simulink model "Full_quadcopter_GR"  (Simulink 7.7)
settings: Solver=ode45  StartTime=0.0  StopTime=10.0  RelTol=1e-3
values from neighbouring files (symbols this model uses):
  b = 9.7575e-6    (= 9.7575e-06)    [ForcesTest.m]    (also in QuadDynamics.m = 9.937e-09; QuadDynamicsC.m = 1.7246e-06; Quadparameters.m = 3.13e-05; quadparam.m = 3.13e-05)
  g = 9.81    [ForcesTest.m]    (also in QuadDynamics.m; QuadDynamicsC.m; Quadparameters.m; quadparam.m)
  k = k+1    (= 1)    [ForcesTest.m]    (also in QuadDynamics.m = 3.82192307692e-10; QuadDynamicsC.m = 6.633e-08)
  m = 1.282    [ForcesTest.m]    (also in QuadDynamics.m = 1.284; QuadDynamicsC.m = 1.284; Quadparameters.m = 0.65; quadparam.m = 0.65)
undefined symbols (not defined in the file or in its folder): r1, r2
settings Model: Creator=Alexey  LastModifiedBy=Alexey

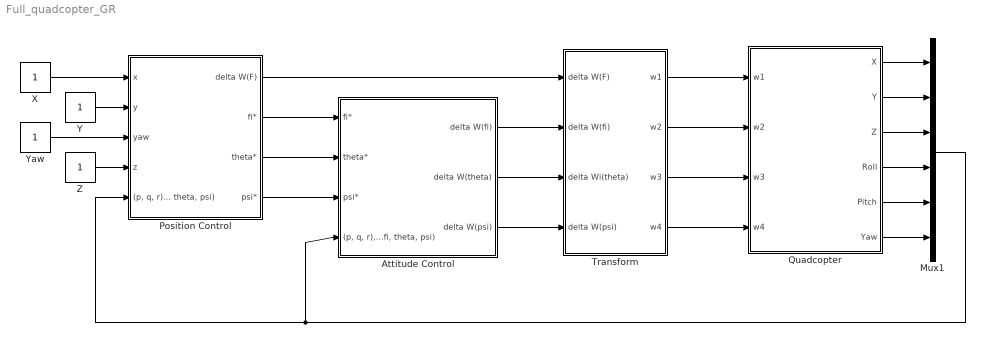
== system Full_quadcopter_GR ==
  Attitude Control : Subsystem
  Mux1 : Mux  Inputs=6
  Position Control : Subsystem
  Quadcopter : Subsystem
  Transform : Subsystem
  X : Constant
  Y : Constant
  Yaw : Constant
  Z : Constant
  wires:
  X/1 -> Position Control/1(x)
  Mux1/1 -> Attitude Control/4("(p, q, r), (fi, theta, psi)"), Position Control/5("(p, q, r), (fi, theta, psi)")
  Quadcopter/1(X) -> Mux1/1
  Quadcopter/2(Y) -> Mux1/2
  Quadcopter/3(Z) -> Mux1/3
  Transform/1(w1) -> Quadcopter/1(w1)
  Transform/2(w2) -> Quadcopter/2(w2)
  Transform/3(w3) -> Quadcopter/3(w3)
  Transform/4(w4) -> Quadcopter/4(w4)
  Position Control/1(delta W(F)) -> Transform/1(delta W(F))
  Attitude Control/1(delta W(fi)) -> Transform/2(delta W(fi))
  Attitude Control/2(delta W(theta)) -> Transform/3(delta Wi(theta))
  Attitude Control/3(delta W(psi)) -> Transform/4(delta W(psi))
  Position Control/2(fi*) -> Attitude Control/1(fi*)
  Position Control/3(theta*) -> Attitude Control/2(theta*)
  Position Control/4(psi*) -> Attitude Control/3(psi*)
  Y/1 -> Position Control/2(y)
  Yaw/1 -> Position Control/3(yaw)
  Z/1 -> Position Control/4(z)
  Quadcopter/4(Roll) -> Mux1/4
  Quadcopter/5(Pitch) -> Mux1/5
  Quadcopter/6(Yaw) -> Mux1/6

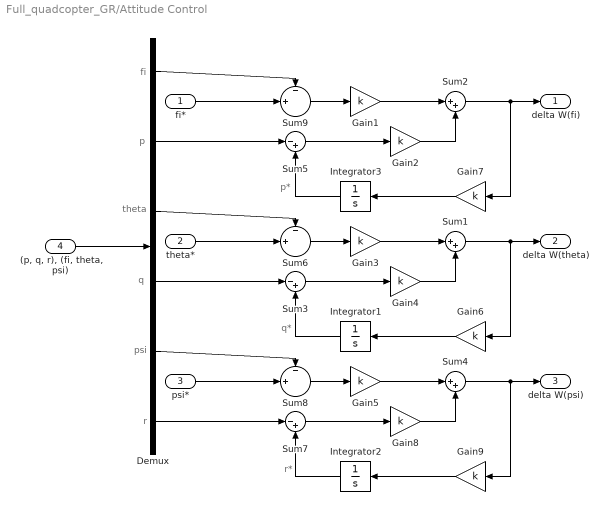
== system Full_quadcopter_GR/Attitude Control ==
  note: fi
  note: p
  note: theta
  note: q
  note: psi
  note: r
  note: q*
  note: p*
  note: r*
  fi* : Inport
  theta* : Inport  Port=2
  psi* : Inport  Port=3
  "(p, q, r), (fi, theta, psi)" : Inport  Port=4
  Demux : Demux  Outputs=6
  Gain{1..9} (9 alike) : Gain  Gain=k
  Integrator1 : Integrator
  Integrator2 : Integrator
  Integrator3 : Integrator
  Sum1 : Sum  Inputs=|++
  Sum2 : Sum  Inputs=|++
  Sum3 : Sum  Inputs=|-+
  Sum4 : Sum  Inputs=|++
  Sum5 : Sum  Inputs=|-+
  Sum6 : Sum  Inputs=-|+||
  Sum7 : Sum  Inputs=|-+
  Sum8 : Sum  Inputs=-|+||
  Sum9 : Sum  Inputs=-|+||
  delta W(fi) : Outport
  delta W(theta) : Outport  Port=2
  delta W(psi) : Outport  Port=3
  wires:
  psi*/1 -> Sum8/2
  Sum8/1 -> Gain5/1
  Gain5/1 -> Sum4/1
  "(p, q, r), (fi, theta, psi)"/1 -> Demux/1
  Sum7/1 -> Gain8/1
  Gain8/1 -> Sum4/2
  Gain9/1 -> Integrator2/1
  Integrator2/1 -> Sum7/2
  Demux/6 -> Sum7/1
  Demux/5 -> Sum8/1
  Sum4/1 -> delta W(psi)/1, Gain9/1
  theta*/1 -> Sum6/2
  Sum6/1 -> Gain3/1
  Gain3/1 -> Sum1/1
  Sum3/1 -> Gain4/1
  Gain4/1 -> Sum1/2
  Gain6/1 -> Integrator1/1
  Integrator1/1 -> Sum3/2
  Demux/4 -> Sum3/1
  Demux/3 -> Sum6/1
  Sum1/1 -> Gain6/1, delta W(theta)/1
  fi*/1 -> Sum9/2
  Sum9/1 -> Gain1/1
  Gain1/1 -> Sum2/1
  Sum5/1 -> Gain2/1
  Gain2/1 -> Sum2/2
  Gain7/1 -> Integrator3/1
  Integrator3/1 -> Sum5/2
  Demux/2 -> Sum5/1
  Demux/1 -> Sum9/1
  Sum2/1 -> Gain7/1, delta W(fi)/1

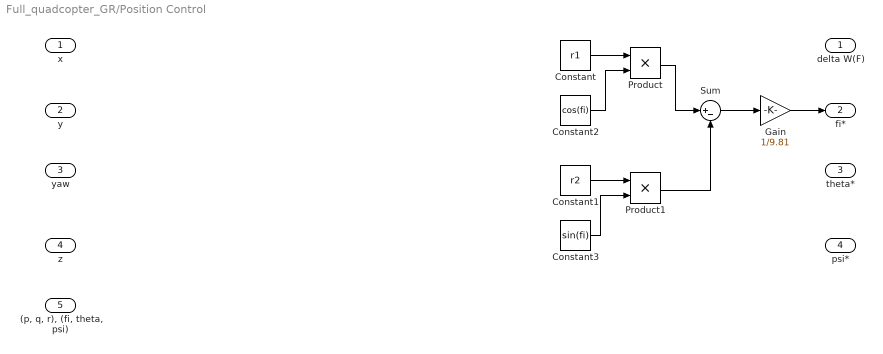
== system Full_quadcopter_GR/Position Control ==
  x : Inport
  y : Inport  Port=2
  yaw : Inport  Port=3
  z : Inport  Port=4
  "(p, q, r), (fi, theta, psi)" : Inport  Port=5
  Constant : Constant  Value=r1
  Constant1 : Constant  Value=r2
  Constant2 : Constant  Value=cos(fi)
  Constant3 : Constant  Value=sin(fi)
  Gain : Gain  Gain=1/9.81
  Product : Product  RndMeth=Zero
  Product1 : Product  RndMeth=Zero
  Sum : Sum  Inputs=|+-
  delta W(F) : Outport
  fi* : Outport  Port=2
  theta* : Outport  Port=3
  psi* : Outport  Port=4
  wires:
  Gain/1 -> fi*/1
  Product/1 -> Sum/1
  Constant/1 -> Product/1
  Constant2/1 -> Product/2
  Constant1/1 -> Product1/1
  Constant3/1 -> Product1/2
  Product1/1 -> Sum/2
  Sum/1 -> Gain/1

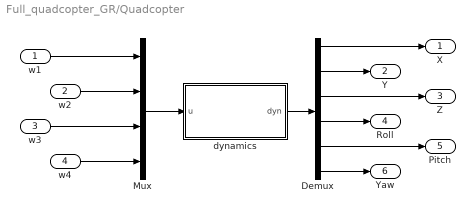
== system Full_quadcopter_GR/Quadcopter ==
  w1 : Inport
  w2 : Inport  Port=2
  w3 : Inport  Port=3
  w4 : Inport  Port=4
  Demux : Demux  Outputs=6
  Mux : Mux
  dynamics : Stateflow chart  TreatAsAtomicUnit=on
  X : Outport
  Y : Outport  Port=2
  Z : Outport  Port=3
  Roll : Outport  Port=4
  Pitch : Outport  Port=5
  Yaw : Outport  Port=6
  wires:
  w1/1 -> Mux/1
  w2/1 -> Mux/2
  w3/1 -> Mux/3
  w4/1 -> Mux/4
  Demux/1 -> X/1
  Demux/2 -> Y/1
  Demux/3 -> Z/1
  Demux/4 -> Roll/1
  Demux/5 -> Pitch/1
  Demux/6 -> Yaw/1
  Mux/1 -> dynamics/1(u)
  dynamics/1(dyn) -> Demux/1

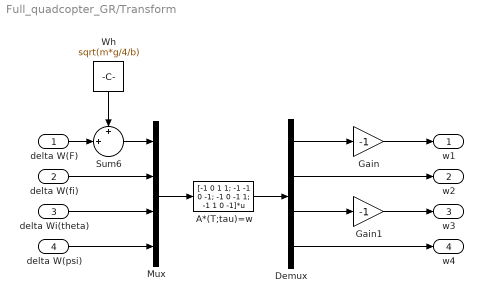
== system Full_quadcopter_GR/Transform ==
  delta W(F) : Inport
  delta W(fi) : Inport  Port=2
  delta Wi(theta) : Inport  Port=3
  delta W(psi) : Inport  Port=4
  A*(T;tau)=w : Fcn  Expr=[-1 0 1 1; -1 -1 0 -1; -1 0 -1 1; -1 1 0 -1]*u
  Demux : Demux
  Gain : Gain  Gain=-1
  Gain1 : Gain  Gain=-1
  Mux : Mux
  Sum6 : Sum  Inputs=+|+||
  Wh : Constant  Value=sqrt(m*g/4/b)
  w1 : Outport
  w2 : Outport  Port=2
  w3 : Outport  Port=3
  w4 : Outport  Port=4
  wires:
  A*(T;tau)=w/1 -> Demux/1
  Mux/1 -> A*(T;tau)=w/1
  Demux/1 -> Gain/1
  Demux/2 -> w2/1
  Demux/3 -> Gain1/1
  Demux/4 -> w4/1
  Gain/1 -> w1/1
  Gain1/1 -> w3/1
  delta W(fi)/1 -> Mux/2
  delta Wi(theta)/1 -> Mux/3
  delta W(psi)/1 -> Mux/4
  delta W(F)/1 -> Sum6/2
  Sum6/1 -> Mux/1
  Wh/1 -> Sum6/1

== matlab function Quadcopter/dynamics ==
  data: u input double; dyn output double
function dyn = quad_dynamics(u)
w = u(1:4);

l=0.3;
h=0.007;
b=0.001;
k=0.001;
m=1;
g=9.81;

Ixx = 0;
Iyy = 0;
Izz = 0;
J = diag([Ixx Iyy Izz]);

D(:,1) = [l;0;h];
D(:,2) = [0;l;h];
D(:,3) = [-l;0;h];
D(:,4) = [0;-l;h];

Rr = [cos(Theta)*cos(Phi)          sin(Psi)*sin(Theta)*cos(Phi)-cos(Psi)*sin(Phi)          cos(Psi)*sin(Theta)*cos(Phi)+sin(Psi)*sin(Phi);
    cos(Theta)*sin(Phi)          sin(Psi)*sin(Theta)*sin(Phi)+cos(Psi)*cos(Phi)           cos(Psi)*sin(Theta)*sin(Phi)-sin(Psi)*cos(Phi);
    -sin(Theta)         sin(Psi)*cos(Theta)        cos(Psi)*cos(Theta)];

OmegaToTheta = (1/cos(Theta))*[0        sin(Psi)          cos(Psi);             
    0        cos(Psi)*cos(Theta)       -sin(Psi)*cos(Theta);
    cos(Theta)      sin(Psi)*sin(Theta)      cos(Psi)*sin(Theta)];

for i=1:4
 T(i) = b * w(i)^2 * [0;0;1];  
 Q(i) = k * w(i)^2 * [0;0;1];    
 tau(i) = cross(T(i),D(i));   
end

dXYZ = Velocity;
dTheta = OmegaToTheta*Omega;

dVelocity = g * [0;0;1] + Rr * (1 / m) * T(i);
dOmega = (cross(-o,J*o) + tau(i)) / J; 

dyn = [dXYZ; dTheta; dVelocity; dOmega];   
end
